simulink model "sim_bloc"  (R2023a)
settings: Solver=VariableStepAuto  StartTime=0.0  StopTime=10.0  RelTol=1e-3
libraries: lib_robotRP_new x2
settings Model: Creator=gbl3344a  LastModifiedBy=gbl3344a

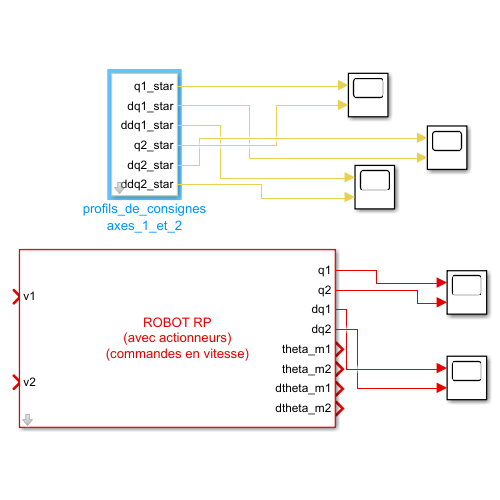
[thumbnail: Simulink's stored preview of the top-level diagram]
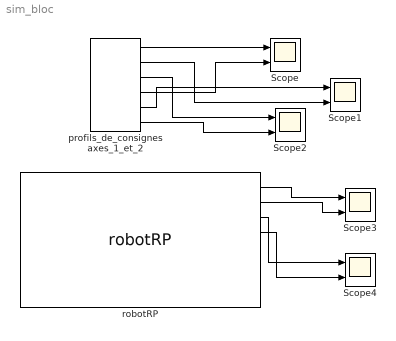
== system sim_bloc ==
  Scope{,1..4} (5 alike) : Scope  NumInputPorts=2
  profils_de_consignes axes_1_et_2 : lib_robotRP_new/profils_de_consignes axes_1_et_2
  robotRP : lib_robotRP_new/robotRP  vecteur_theta_dtheta_initial=[0 ; 100 ; 0 ; 0]  m=15  gX=0  gY=-9.81  F1=0  F2=0  H1=0  H2=0  Km_sur_R=0.3  Jm=0.01  Beff=0.0125  r=1/30
  wires:
  profils_de_consignes axes_1_et_2/1 -> Scope/1
  profils_de_consignes axes_1_et_2/4 -> Scope/2
  profils_de_consignes axes_1_et_2/5 -> Scope1/1
  profils_de_consignes axes_1_et_2/2 -> Scope1/2
  profils_de_consignes axes_1_et_2/3 -> Scope2/1
  profils_de_consignes axes_1_et_2/6 -> Scope2/2
  robotRP/1 -> Scope3/1
  robotRP/2 -> Scope3/2
  robotRP/3 -> Scope4/1
  robotRP/4 -> Scope4/2
